simulink model "CML_Iso_Force_Production"  (R2015a)
settings: Solver=ode4  SolverMode=MultiTasking  StartTime=0.0  StopTime=inf  FixedStep=BKIN_STEP_TIME  RelTol=1e-3
StartFcn:
  |  warndlg('Dexterit-E models cannot run under simulation. Please compile your model and run it from within Dexterit-E.');set_param(bdroot,'SimulationCommand','stop')
model workspace (MAT data in the model file):
  BKIN_STEP_TIME = 0.00025
  col_x = 1
  col_y = 2
  VRAD = 3
  COLOR = 4
  TARGET_COL = 2
  BKIN_KINEMATIC_FRAME_SIZE = 400
  E_NO_EVENT = 0
  K_START_TGT = 1
  INIT_DUR = 5
  TP_ITI = 9
  K_JOINT_ASSESSED = 2
  TEXT1 = 5
  TEXT2 = 6
  HEIGHT = 7
  STROKE_WIDTH = 8
  GOAL_F_PCT = 3
  DO_FDBK = 8
  MAX_MOVE_TIME = 7
  MIN_FORCE = 4
  E_TEST_MVC = 1
  E_HOLD_MVC = 3
  E_EOT = 10
  E_FORCE_TRIAL = 11
  E_HOLD_FORCE = 13
  K_BAR_TGT = 3
  K_MVC_TEXT_TGT = 4
  E_INIT_FORCE = 12
  E_SET_MVC = 2
  K_MVC = 5
  TRIAL_TYPE = 1
  HOLD_TIME = 6
  E_ERROR_TRIAL = 5
  E_ACCEPT_MVC = 6
  ACCEPT_MVC = 2
  REJECT_MVC = 3
  E_CHECK_MVC = 4
  E_REJECT_MVC = 5
libraries: Video x5, slrtlib x5, General x3, KINARM_IO x2, simulink x2, KINARM_loads x2, KINARM_general x1, xpcnilib x1
CloseFcn:
  | rtwprivate ssgencode ModelCloseRequest b2lab2d
settings Model: ModifiedComment=chris -- Wed Feb 16 09:18:30 2005 -- Version 1.1384  ExtModeArmWhenConnect=off  ExtModeLogAll=off  LastModifiedBy=User
settings SolverCC: EnableConcurrentExecution=on  AutoInsertRateTranBlk=on
settings DataIOCC: LimitDataPoints=off  SignalLoggingSaveFormat=ModelDataLogs  SaveOutput=off  SaveTime=off  SignalLoggingName=sigsOut
settings OptimizationCC: BlockReduction=off  BooleanDataType=off  OptimizeBlockIOStorage=off  BufferReuse=off  GlobalBufferReuse=off  ExpressionFolding=off  ExpressionDepthLimit=2147483647  LocalBlockOutputs=off  InitFltsAndDblsToZero=on
settings DebuggingCC: SaveWithParameterizedLinksMsg=none  UnderspecifiedInitializationDetection=Classic  MergeDetectMultiDrivingBlocksExec=none  SignalResolutionControl=TryResolveAllWithWarning  MultiTaskDSMMsg=warning  FcnCallInpInsideContextMsg=UseLocalSettings  StateNameClashWarn=warning  StrictBusMsg=ErrorOnBusTreatedAsVector
settings HardwareCC: ProdIntDivRoundTo=Zero  ProdEndianess=LittleEndian  ProdLongLongMode=on  ProdHWDeviceType=Generic->32-bit x86 compatible  TargetHWDeviceType=32-bit Generic
settings SFSimCC: SimParseCustomCode=off
settings RTWCC: SystemTargetFile=slrt.tlc  TemplateMakefile=slrt_default_tmf  Description=Simulink Real-Time  RTWCompilerOptimization=on
settings CodeAppCC: MaxIdLength=63
settings SimulinkRealTimeCC: TargetFcnLib=ansi_tfl_tmw.mat  GeneratePreprocessorConditionals=Disable all  xPCisDownloadable=off

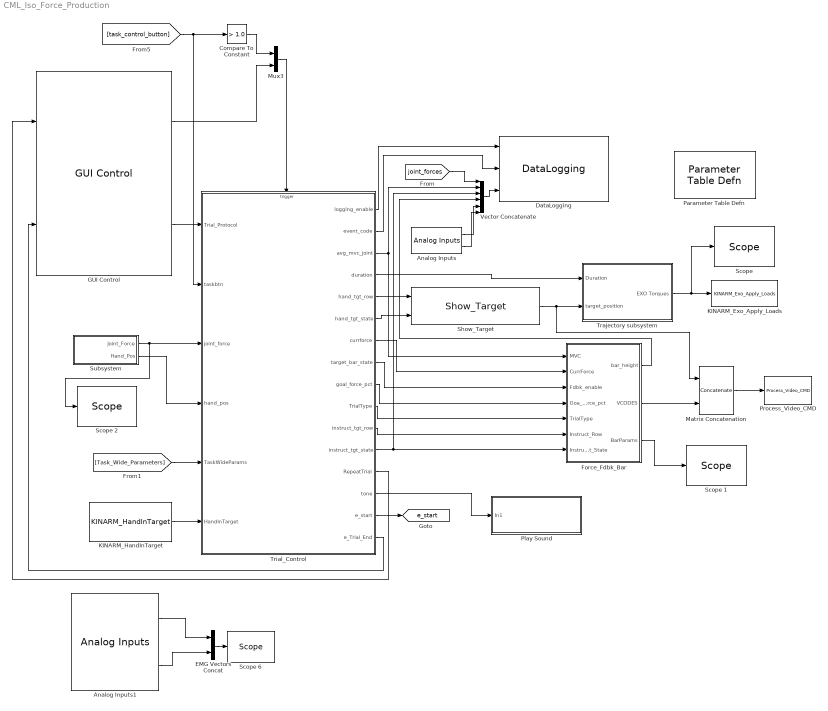
== system CML_Iso_Force_Production ==
  Analog Inputs : KINARM_IO/Analog Inputs  channel=[18:19]  range=[5]  coupling=[0]  scantime6071e=1.28e-5  scantime6229=5e-6  sampletime=0.001  slot=-1  oscantime6071e=0
  Analog Inputs1 : KINARM_IO/Analog Inputs  channel=[18:19]  range=[5]  coupling=[0]  scantime6071e=1.28e-5  scantime6229=5e-6  sampletime=0.001  slot=-1  oscantime6071e=0
  Compare To Constant : simulink/Logic and Bit Operations/Compare To Constant  relop=>  const=1.0  OutDataTypeStr=boolean
  DataLogging : General/DataLogging  log_event_codes=on  log_analog_inputs=on  show_time_remaining=off  ecat_include=on
      link override Poll KINARM/EPTorqueCMD: GotoTag=KINARMEPTorqueCMD
      link override Poll KINARM/TorqueCMD: GotoTag=KINARMTorqueCMD
  EMG Vectors Concat : Concatenate
  Force_Fdbk_Bar : Subsystem
  GUI Control : General/GUI Control  task_version=1.0  show_repeat_trial_flag=on  use_custom_tp=off  target_type_str=Circle  Target_Type=1  XYcols=[1 2]  Vcols=3  Lcols=4  indices_padding=[0 0 0 0;0 0 0 0]  target_table_rows=64  load_table_rows=20  tp_table_rows=100
  KINARM_Exo_Apply_Loads : KINARM_loads/KINARM_Exo_Apply_Loads  up_duration=1000  down_duration=1000  max_torque=10  limit_motors=off
  KINARM_HandInTarget : KINARM_general/KINARM_HandInTarget  use_dominant_hand=on  target_type=Circle  num_states=1  attribcol1=[VRAD]  attribcol2=[0]  attribcol3=[0]  attribcol4=[0]  attribcol5=[0]
  Matrix Concatenation : Concatenate  Mode=Multidimensional array
  Mux3 : Mux  Inputs=2
  Parameter Table Defn : General/Parameter Table Defn  ShowInLibBrowser=0
  Play Sound : Subsystem
  Process_Video_CMD : Video/Process_Video_CMD  video_delay=0
  "Scope " : slrtlib/Displays and Logging/Scope   scopeno=1  scopetype=Target  autostart=on  viewmode=Numerical  formatstr='%15.6f'  grid=on  ylimits=[0,0]  nosamples=250  noprepostsamples=0  interleave=1  triggermode=FreeRun  triggersignal=1  trigsignalfromport=off  triggerlevel=0.0  triggerslope=Either  triggerscope=1  triggersample=0  filename=data.dat  mode=Lazy  writesize=512  autorestart=off  dynamicfilemode=off  maxwritefilesize=512*1024^2
  Scope 1 : slrtlib/Displays and Logging/Scope   scopeno=2  scopetype=Target  autostart=on  viewmode=Numerical  formatstr='%15.6f'  grid=on  ylimits=[0,0]  nosamples=250  noprepostsamples=0  interleave=1  triggermode=FreeRun  triggersignal=1  trigsignalfromport=off  triggerlevel=0.0  triggerslope=Either  triggerscope=1  triggersample=0  filename=data.dat  mode=Lazy  writesize=512  autorestart=off  dynamicfilemode=off  maxwritefilesize=512*1024^2
  Scope 2 : slrtlib/Displays and Logging/Scope   scopeno=3  scopetype=Target  autostart=on  viewmode=Numerical  formatstr='%15.6f'  grid=on  ylimits=[0,0]  nosamples=250  noprepostsamples=0  interleave=1  triggermode=FreeRun  triggersignal=1  trigsignalfromport=off  triggerlevel=0.0  triggerslope=Either  triggerscope=1  triggersample=0  filename=data.dat  mode=Lazy  writesize=512  autorestart=off  dynamicfilemode=off  maxwritefilesize=512*1024^2
  Scope 6 : slrtlib/Displays and Logging/Scope   scopeno=4  scopetype=Target  autostart=on  viewmode=Numerical  formatstr='%15.6f'  grid=on  ylimits=[0,0]  nosamples=250  noprepostsamples=0  interleave=1  triggermode=FreeRun  triggersignal=1  trigsignalfromport=off  triggerlevel=0.0  triggerslope=Either  triggerscope=1  triggersample=0  filename=data.dat  mode=Lazy  writesize=512  autorestart=off  dynamicfilemode=off  maxwritefilesize=512*1024^2
  Show_Target : Video/Show_Target  target_type=Circle  num_states=1  attribcol1=[COLOR 0 0 VRAD]  attribcol2=[0 0 0 0]  attribcol3=[0 0 0 0]  attribcol4=[0 0 0 0]  attribcol5=[0 0 0 0]  stateindices_padding=[0 0 0 0 0 0 0;0 0 0 0 0 0 0;0 0 0 0 0 0 0;0 0 0 0 0 0 0;0 0 0 0 0 0 0]  source=dialog  opacity=100  target_display=Both subject and operator displays  num_col=4
  Subsystem : Subsystem
  Trajectory subsystem : Subsystem
  Trial_Control : Stateflow chart  TreatAsAtomicUnit=on
  Vector Concatenate : Concatenate  NumInputs=6
  tag scope: e_start=global
  wires:
  Show_Target/1 -> Matrix Concatenation/1, Trajectory subsystem/2(target_position)
  Trial_Control/16(e_Trial_End) -> GUI Control/2
  GUI Control/1 -> Mux3/2
  Trial_Control/6(hand_tgt_state) -> Show_Target/2
  Trial_Control/5(hand_tgt_row) -> Show_Target/1
  Matrix Concatenation/1 -> Process_Video_CMD/1
  GUI Control/2 -> Trial_Control/1(Trial_Protocol)
  Trial_Control/1(logging_enable) -> DataLogging/1
  Trial_Control/4(duration) -> Trajectory subsystem/1(Duration)
  Trajectory subsystem/1(EXO Torques) -> "Scope "/1, KINARM_Exo_Apply_Loads/1
  Trial_Control/15(e_start) -> [e_start]
  [joint_forces] -> Vector Concatenate/1
  Vector Concatenate/1 -> DataLogging/3
  Analog Inputs/1 -> Vector Concatenate/5
  Subsystem/1(Joint_Force) -> Scope 2/1, Trial_Control/3(joint_force)
  Subsystem/2(Hand_Pos) -> Trial_Control/4(hand_pos)
  [Task_Wide_Parameters] -> Trial_Control/5(TaskWideParams)
  Trial_Control/11(instruct_tgt_row) -> Force_Fdbk_Bar/6(Instruct_Row)
  Trial_Control/12(instruct_tgt_state) -> Force_Fdbk_Bar/7(Instruct_State), Vector Concatenate/3
  Trial_Control/3(avg_mvc_joint) -> Force_Fdbk_Bar/1(MVC), Vector Concatenate/2
  Force_Fdbk_Bar/2(VCODES) -> Matrix Concatenation/2
  Trial_Control/8(target_bar_state) -> Force_Fdbk_Bar/3(Fdbk_enable)
  Trial_Control/7(currforce) -> Force_Fdbk_Bar/2(CurrForce)
  Trial_Control/9(goal_force_pct) -> Force_Fdbk_Bar/4(Goa_force_pct)
  Force_Fdbk_Bar/1(bar_height) -> Vector Concatenate/4
  Force_Fdbk_Bar/3(BarParams) -> Scope 1/1
  Trial_Control/2(event_code) -> DataLogging/2
  Trial_Control/10(TrialType) -> Force_Fdbk_Bar/5(TrialType)
  KINARM_HandInTarget/1 -> Trial_Control/6(HandInTarget)
  Trial_Control/14(tone) -> Play Sound/1(In1)
  Trial_Control/13(RepeatTrial) -> GUI Control/1
  [task_control_button] -> Compare To Constant/1, Trial_Control/2(taskbtn)
  Compare To Constant/1 -> Mux3/1
  Mux3/1 -> Trial_Control/Trigger
  EMG Vectors Concat/1 -> Scope 6/1
  Analog Inputs1/1 -> EMG Vectors Concat/1
  Analog Inputs1/2 -> EMG Vectors Concat/2
  Analog Inputs/2 -> Vector Concatenate/6

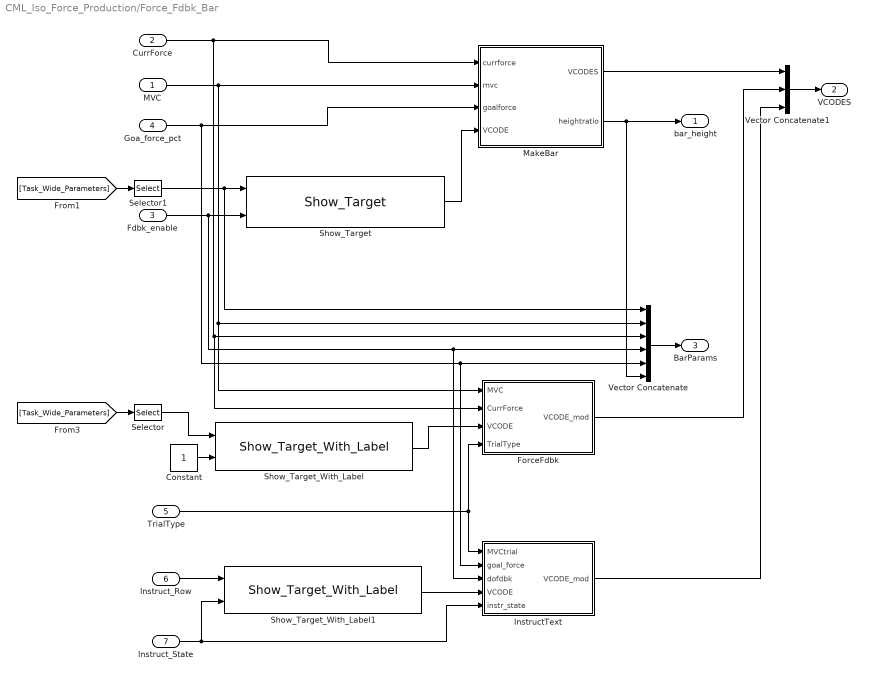
== system CML_Iso_Force_Production/Force_Fdbk_Bar ==
  MVC : Inport
  CurrForce : Inport  Port=2
  Fdbk_enable : Inport  Port=3
  Goa_force_pct : Inport  Port=4
  TrialType : Inport  Port=5
  Instruct_Row : Inport  Port=6
  Instruct_State : Inport  Port=7
  Constant : Constant
  ForceFdbk : MATLAB Function  TreatAsAtomicUnit=on
  InstructText : MATLAB Function  TreatAsAtomicUnit=on
  MakeBar : MATLAB Function  TreatAsAtomicUnit=on
  Selector : Selector  InputPortWidth=50  Indices=[K_MVC_TEXT_TGT]
  Selector1 : Selector  InputPortWidth=50  Indices=[K_BAR_TGT]
  Show_Target : Video/Show_Target  target_type=Rectangle  num_states=1  attribcol1=[COLOR 0 STROKE_WIDTH VRAD HEIGHT 0]  attribcol2=[0 0 0 0 0 0]  attribcol3=[0 0 0 0 0 0]  attribcol4=[0 0 0 0 0 0]  attribcol5=[0 0 0 0 0 0]  stateindices_padding=[0 0 0 0 0;0 0 0 0 0;0 0 0 0 0;0 0 0 0 0;0 0 0 0 0]  source=dialog  opacity=100  target_display=Both subject and operator displays  num_col=6
  Show_Target_With_Label : Video/Show_Target_With_Label  target_type=Rectangle  num_states=1  attribcol1=[0 0 0 VRAD HEIGHT 0 TEXT1 COLOR HEIGHT]  attribcol2=[0 0 0 0 0 0 0 0 0]  attribcol3=[0 0 0 0 0 0 0 0 0]  attribcol4=[0 0 0 0 0 0 0 0 0]  attribcol5=[0 0 0 0 0 0 0 0 0]  stateindices_padding=[0 0;0 0;0 0;0 0;0 0]  source=dialog  opacity=100  target_display=Operator display only
  Show_Target_With_Label1 : Video/Show_Target_With_Label  target_type=Rectangle  num_states=2  attribcol1=[0 0 0 VRAD HEIGHT 0 TEXT1 COLOR HEIGHT]  attribcol2=[0 0 0 VRAD HEIGHT 0 TEXT2 COLOR HEIGHT]  attribcol3=[0 0 0 0 0 0 0 0 0]  attribcol4=[0 0 0 0 0 0 0 0 0]  attribcol5=[0 0 0 0 0 0 0 0 0]  stateindices_padding=[0 0;0 0;0 0;0 0;0 0]  source=dialog  opacity=100  target_display=Both subject and operator displays
  Vector Concatenate : Concatenate  NumInputs=6
  Vector Concatenate1 : Concatenate  NumInputs=3  Mode=Multidimensional array
  bar_height : Outport
  VCODES : Outport  Port=2
  BarParams : Outport  Port=3
  wires:
  Fdbk_enable/1 -> InstructText/3(dofdbk), Vector Concatenate/4, Show_Target/2
  Selector1/1 -> Vector Concatenate/1, Show_Target/1
  CurrForce/1 -> ForceFdbk/2(CurrForce), Vector Concatenate/3, MakeBar/1(currforce)
  MVC/1 -> ForceFdbk/1(MVC), Vector Concatenate/2, MakeBar/2(mvc)
  Show_Target/1 -> MakeBar/4(VCODE)
  MakeBar/1(VCODES) -> Vector Concatenate1/1
  Goa_force_pct/1 -> Vector Concatenate/5, InstructText/2(goal_force), MakeBar/3(goalforce)
  MakeBar/2(heightratio) -> Vector Concatenate/6, bar_height/1
  Vector Concatenate/1 -> BarParams/1
  Constant/1 -> Show_Target_With_Label/2
  Show_Target_With_Label/1 -> ForceFdbk/3(VCODE)
  ForceFdbk/1(VCODE_mod) -> Vector Concatenate1/2
  Vector Concatenate1/1 -> VCODES/1
  TrialType/1 -> ForceFdbk/4(TrialType), InstructText/1(MVCtrial)
  Selector/1 -> Show_Target_With_Label/1
  [Task_Wide_Parameters] -> Selector/1
  Show_Target_With_Label1/1 -> InstructText/4(VCODE)
  Instruct_Row/1 -> Show_Target_With_Label1/1
  Instruct_State/1 -> InstructText/5(instr_state), Show_Target_With_Label1/2
  InstructText/1(VCODE_mod) -> Vector Concatenate1/3
  [Task_Wide_Parameters] -> Selector1/1

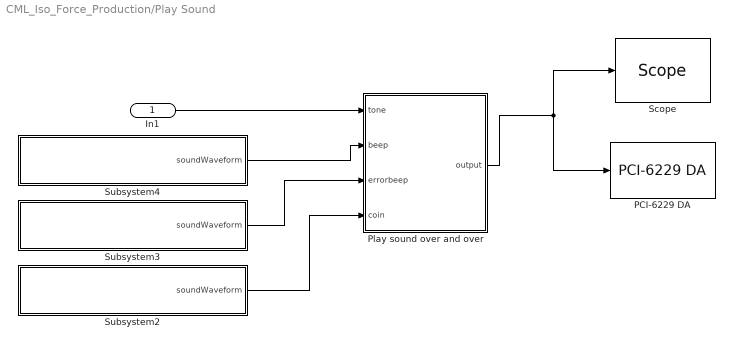
== system CML_Iso_Force_Production/Play Sound ==
  In1 : Inport
  PCI-6229 DA : xpcnilib/D//A/M Series/PCI-6229 DA  channel=[1]  reset=[1]  initValue=[0]  sampletime=-1  slot=-1
  Play sound over and over : MATLAB Function  TreatAsAtomicUnit=on
  "Scope " : slrtlib/Displays and Logging/Scope   scopeno=5  scopetype=Target  autostart=on  viewmode=Graphical redraw  formatstr='%15.6f'  grid=on  ylimits=[0,0]  nosamples=4000  noprepostsamples=0  interleave=1  triggermode=FreeRun  triggersignal=1  trigsignalfromport=off  triggerlevel=0.0  triggerslope=Either  triggerscope=1  triggersample=0  filename=data.dat  mode=Lazy  writesize=512  autorestart=off  dynamicfilemode=off  maxwritefilesize=512*1024^2
  Subsystem2 : Subsystem  mask(Load Waveform Into Variable){fileName=coin.mat}
      mask prompts: fileName "Name of .mat Data File (must be in current directory)"
      mask help: This block will load the .MAT file specified in the dialog, and put the first variable into a GoTo called 'soundWaveform'.
      mask init:
      | filenameFromMask = get_param(gcb, 'fileName');
      | 
      | try 
      | 	dataFromFile = load(filenameFromMask);
      | 	names = fieldnames(dataFromFile);
      | 	soundDataFromFile = dataFromFile.(names{1});
      | 	display(['Sound waveform from file ''' filenameFromMask ''' loaded.']);
      | catch ME
      | 	display(ME.message)
      | end
      mask Help:
      | Enter the name a .MAT file containing a single vector or matrix. The .MAT file must be located in the current directory.
      | 
      | The first variable from the .MAT file will be put into a Goto called 'soundWaveform'.
      mask Display: disp(['Load waveform from ''' filenameFromMask ''''])
  Subsystem3 : Subsystem  mask(Load Waveform Into Variable){fileName=errorbeep.mat}
      mask prompts: fileName "Name of .mat Data File (must be in current directory)"
      mask help: This block will load the .MAT file specified in the dialog, and put the first variable into a GoTo called 'soundWaveform'.
      mask init: same as CML_Iso_Force_Production/Play Sound/Subsystem2
      mask Help:
      | Enter the name a .MAT file containing a single vector or matrix. The .MAT file must be located in the current directory.
      | 
      | The first variable from the .MAT file will be put into a Goto called 'soundWaveform'.
      mask Display: disp(['Load waveform from ''' filenameFromMask ''''])
  Subsystem4 : Subsystem  mask(Load Waveform Into Variable){fileName=startbeep.mat}
      mask prompts: fileName "Name of .mat Data File (must be in current directory)"
      mask help: This block will load the .MAT file specified in the dialog, and put the first variable into a GoTo called 'soundWaveform'.
      mask init: same as CML_Iso_Force_Production/Play Sound/Subsystem2
      mask Help:
      | Enter the name a .MAT file containing a single vector or matrix. The .MAT file must be located in the current directory.
      | 
      | The first variable from the .MAT file will be put into a Goto called 'soundWaveform'.
      mask Display: disp(['Load waveform from ''' filenameFromMask ''''])
  wires:
  Play sound over and over/1(output) -> PCI-6229 DA/1, "Scope "/1
  Subsystem3/1(soundWaveform) -> Play sound over and over/3(errorbeep)
  Subsystem4/1(soundWaveform) -> Play sound over and over/2(beep)
  In1/1 -> Play sound over and over/1(tone)
  Subsystem2/1(soundWaveform) -> Play sound over and over/4(coin)

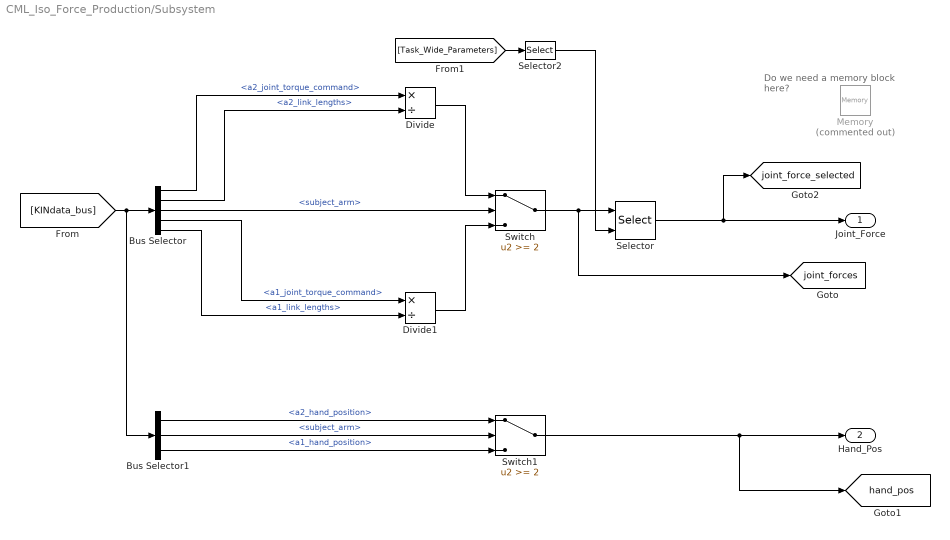
== system CML_Iso_Force_Production/Subsystem ==
  note: Do we need a memory block here?
  Bus Selector : BusSelector  OutputSignals=Robot2.a2_joint_torque_command,Robot2.a2_link_lengths,KINDataGeneral.subject_arm,Robot1.a1_joint_torque_command,Robot1.a1_link_lengths
  Bus Selector1 : BusSelector  OutputSignals=Robot2.a2_hand_position,KINDataGeneral.subject_arm,Robot1.a1_hand_position
  Divide : Product  Inputs=*/
  Divide1 : Product  Inputs=*/
  Memory : Memory  Commented=on
  Selector : Selector  InputPortWidth=2  IndexOptions=Index vector (port)  Indices=[1 3]
  Selector2 : Selector  InputPortWidth=50  Indices=[K_JOINT_ASSESSED]
  Switch : Switch  Threshold=2
  Switch1 : Switch  Threshold=2
  Joint_Force : Outport
  Hand_Pos : Outport  Port=2
  tag scope: hand_pos=global, joint_force_selected=global, joint_forces=global
  wires:
  [KINdata_bus] -> Bus Selector1/1, Bus Selector/1
  Bus Selector/3 -> Switch/2  "<subject_arm>"
  Divide/1 -> Switch/1
  Divide1/1 -> Switch/3
  Bus Selector/1 -> Divide/1  "<a2_joint_torque_command>"
  Bus Selector/2 -> Divide/2  "<a2_link_lengths>"
  Bus Selector/4 -> Divide1/1  "<a1_joint_torque_command>"
  Bus Selector/5 -> Divide1/2  "<a1_link_lengths>"
  Bus Selector1/1 -> Switch1/1  "<a2_hand_position>"
  Bus Selector1/2 -> Switch1/2  "<subject_arm>"
  Bus Selector1/3 -> Switch1/3  "<a1_hand_position>"
  Switch/1 -> Selector/1, [joint_forces]
  Selector2/1 -> Selector/2
  Switch1/1 -> [hand_pos], Hand_Pos/1
  Selector/1 -> [joint_force_selected], Joint_Force/1
  [Task_Wide_Parameters] -> Selector2/1

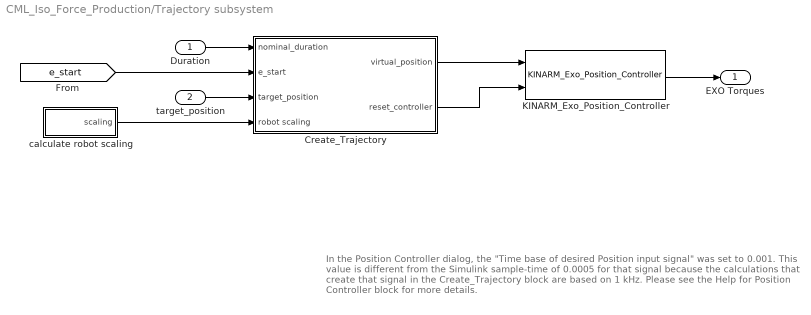
== system CML_Iso_Force_Production/Trajectory subsystem ==
  note: In the Position Controller dialog, the "Time base of desired Position input signal" was set to 0.001.
      | This value is different from the Simulink sample-time of 0.0005 for that signal because the calculations
      | that create that signal in the Create_Trajectory block are based on 1 kHz. Please see the Help for
      | Position Controller block for more details.
  Duration : Inport
  target_position : Inport  Port=2
  Create_Trajectory : Subsystem
  KINARM_Exo_Position_Controller : KINARM_loads/KINARM_Exo_Position_Controller  use_dom_hand=on  KINARM_Type=Human  inertias_for_FF=KINARM robot  angles_or_XY=End-point (global x/y)  sample_time=0.001
  calculate robot scaling : Subsystem
  EXO Torques : Outport
  wires:
  Create_Trajectory/2(reset_controller) -> KINARM_Exo_Position_Controller/2
  Create_Trajectory/1(virtual_position) -> KINARM_Exo_Position_Controller/1
  KINARM_Exo_Position_Controller/1 -> EXO Torques/1
  target_position/1 -> Create_Trajectory/3(target_position)
  Duration/1 -> Create_Trajectory/1(nominal_duration)
  [e_start] -> Create_Trajectory/2(e_start)
  calculate robot scaling/1(scaling) -> Create_Trajectory/4(robot scaling)

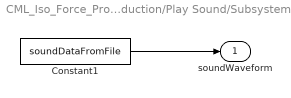
== system CML_Iso_Force_Production/Play Sound/Subsystem2 ==
  Constant1 : Constant  Value=soundDataFromFile
  soundWaveform : Outport
  wires:
  Constant1/1 -> soundWaveform/1

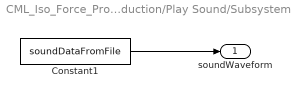
== system CML_Iso_Force_Production/Play Sound/Subsystem3 ==
  Constant1 : Constant  Value=soundDataFromFile
  soundWaveform : Outport
  wires:
  Constant1/1 -> soundWaveform/1

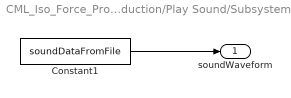
== system CML_Iso_Force_Production/Play Sound/Subsystem4 ==
  Constant1 : Constant  Value=soundDataFromFile
  soundWaveform : Outport
  wires:
  Constant1/1 -> soundWaveform/1

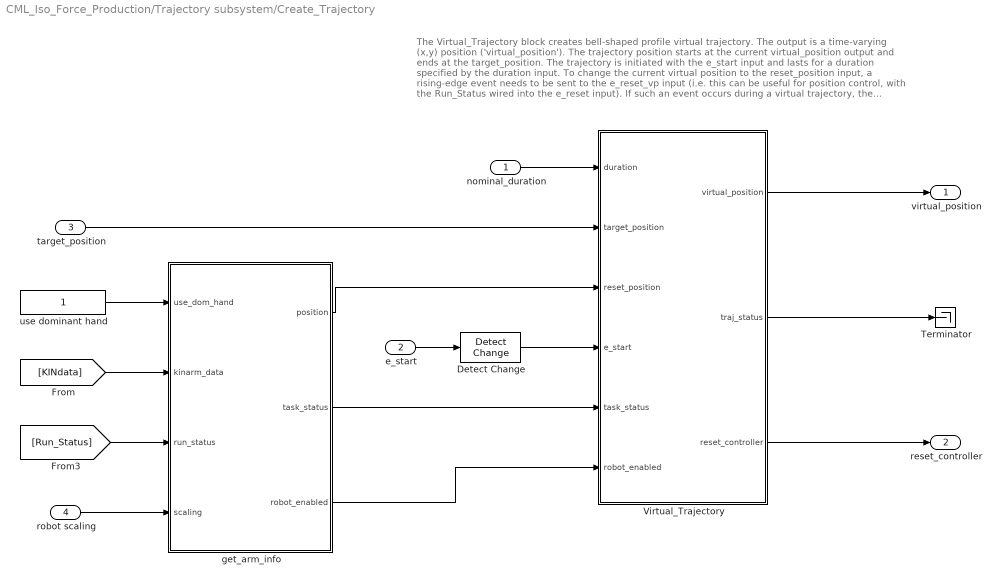
== system CML_Iso_Force_Production/Trajectory subsystem/Create_Trajectory ==
  note: The Virtual_Trajectory block creates bell-shaped profile virtual trajectory.
      | The output is a time-varying (x,y) position ('virtual_position').
      |
      | The trajectory position starts at the current virtual_position output and ends at the target_position.
      | The trajectory is initiated with the e_start input and lasts for a duration specified by the duration input.
      |
      | To change the current virtual position to the reset_position input, a rising-edge event needs to be sent to the e_reset_vp input
      | (i.e. this can be useful for position control, with the Run_Status wired into the e_reset input).
      | If such an event occurs during a virtual trajectory, the trajectory is halted immediately.
  nominal_duration : Inport
  e_start : Inport  Port=2
  target_position : Inport  Port=3
  robot scaling : Inport  Port=4
  Detect Change : simulink/Logic and Bit Operations/Detect Change  vinit=0  InputProcessing=Inherited  OutDataTypeStr=uint8
  Terminator : Terminator
  Virtual_Trajectory : Subsystem
  get_arm_info : MATLAB Function  TreatAsAtomicUnit=on
  use dominant hand : Constant
  virtual_position : Outport
  reset_controller : Outport  Port=2
  wires:
  Virtual_Trajectory/1(virtual_position) -> virtual_position/1
  nominal_duration/1 -> Virtual_Trajectory/1(duration)
  e_start/1 -> Detect Change/1
  target_position/1 -> Virtual_Trajectory/2(target_position)
  Detect Change/1 -> Virtual_Trajectory/4(e_start)
  use dominant hand/1 -> get_arm_info/1(use_dom_hand)
  [KINdata] -> get_arm_info/2(kinarm_data)
  get_arm_info/1(position) -> Virtual_Trajectory/3(reset_position)
  Virtual_Trajectory/3(reset_controller) -> reset_controller/1
  get_arm_info/2(task_status) -> Virtual_Trajectory/5(task_status)
  get_arm_info/3(robot_enabled) -> Virtual_Trajectory/6(robot_enabled)
  [Run_Status] -> get_arm_info/3(run_status)
  Virtual_Trajectory/2(traj_status) -> Terminator/1
  robot scaling/1 -> get_arm_info/4(scaling)

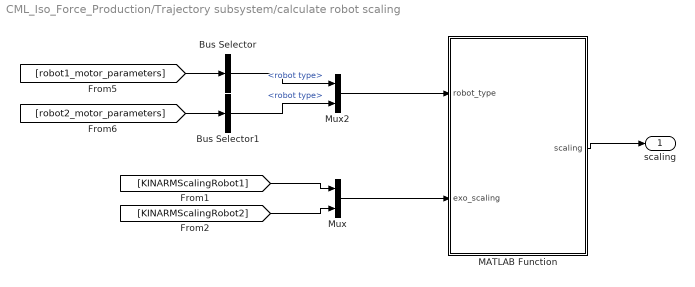
== system CML_Iso_Force_Production/Trajectory subsystem/calculate robot scaling ==
  Bus Selector : BusSelector  OutputSignals=robot type
  Bus Selector1 : BusSelector  OutputSignals=robot type
  MATLAB Function : MATLAB Function  TreatAsAtomicUnit=on
  Mux : Mux  Inputs=2
  Mux2 : Mux  Inputs=2
  scaling : Outport
  wires:
  [KINARMScalingRobot1] -> Mux/1
  [KINARMScalingRobot2] -> Mux/2
  Mux/1 -> MATLAB Function/2(exo_scaling)
  Mux2/1 -> MATLAB Function/1(robot_type)
  MATLAB Function/1(scaling) -> scaling/1
  [robot2_motor_parameters] -> Bus Selector1/1
  Bus Selector1/1 -> Mux2/2  "<robot type>"
  Bus Selector/1 -> Mux2/1  "<robot type>"
  [robot1_motor_parameters] -> Bus Selector/1

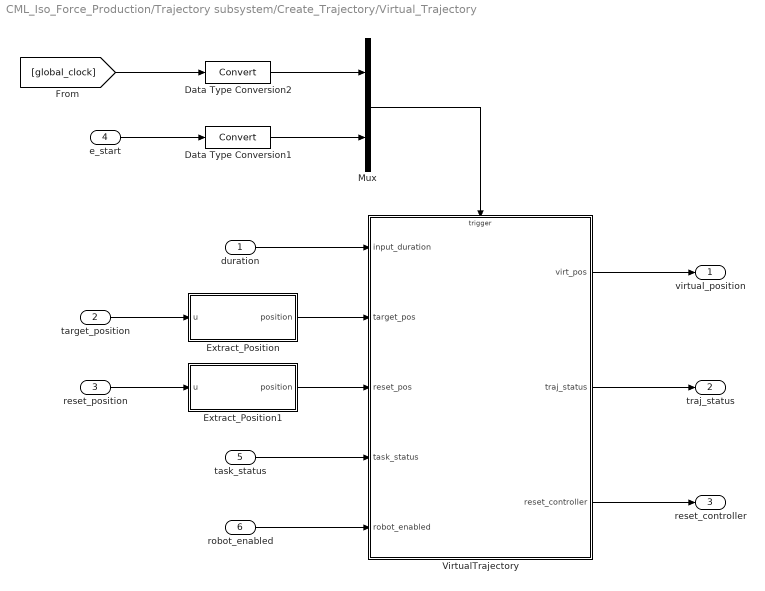
== system CML_Iso_Force_Production/Trajectory subsystem/Create_Trajectory/Virtual_Trajectory ==
  duration : Inport
  target_position : Inport  Port=2
  reset_position : Inport  Port=3
  e_start : Inport  Port=4
  task_status : Inport  Port=5
  robot_enabled : Inport  Port=6
  Data Type Conversion1 : DataTypeConversion
  Data Type Conversion2 : DataTypeConversion
  Extract_Position : MATLAB Function  TreatAsAtomicUnit=on
  Extract_Position1 : MATLAB Function  TreatAsAtomicUnit=on
  Mux : Mux  Inputs=2
  VirtualTrajectory : Stateflow chart  TreatAsAtomicUnit=on
  virtual_position : Outport
  traj_status : Outport  Port=2
  reset_controller : Outport  Port=3
  wires:
  e_start/1 -> Data Type Conversion1/1
  target_position/1 -> Extract_Position/1(u)
  [global_clock] -> Data Type Conversion2/1
  Mux/1 -> VirtualTrajectory/Trigger
  duration/1 -> VirtualTrajectory/1(input_duration)
  VirtualTrajectory/1(virt_pos) -> virtual_position/1
  Extract_Position/1(position) -> VirtualTrajectory/2(target_pos)
  reset_position/1 -> Extract_Position1/1(u)
  Data Type Conversion2/1 -> Mux/1
  VirtualTrajectory/2(traj_status) -> traj_status/1
  robot_enabled/1 -> VirtualTrajectory/5(robot_enabled)
  task_status/1 -> VirtualTrajectory/4(task_status)
  Data Type Conversion1/1 -> Mux/2
  Extract_Position1/1(position) -> VirtualTrajectory/3(reset_pos)
  VirtualTrajectory/3(reset_controller) -> reset_controller/1

== stateflow chart CML_Iso_Force_Production/Trial_Control ==
  settings: sampleTime=0.001
  state init/
    //bring the hand to the start position
    mvc_joint = 0;
    avg_mvc_joint = TaskWideParams[K_MVC];
    n_mvc = 1*(avg_mvc_joint>1e-4);
    hand_tgt_row = TaskWideParams[K_START_TGT];
    hand_tgt_state = 1;
    instruct_tgt_row = 0;
    instruct_tgt_state = 0;
    duration = 3000;
  state MovToStart/
    ITI = Trial_Protocol[TP_ITI];
    TrialType = Trial_Protocol[TRIAL_TYPE];
    RepeatTrial = 0;
    instruct_tgt_state = 0;
    target_bar_state = 0;
    currforce = 0;
    tone = 0;
    e_start;
  state Main_Trial
    state InitMVC/
      event_code = E_TEST_MVC;
      logging_enable = 1;
      duration = 1;
      instruct_tgt_row = Trial_Protocol[TARGET_COL];
      instruct_tgt_state = 1;
      min_force = Trial_Protocol[MIN_FORCE];
      tmpforce = 0;
      tmpcounter = 0;
      iforce = 0;
      maxforce = min_force;
      hold_time = Trial_Protocol[HOLD_TIME];
      max_move_time = Trial_Protocol[MAX_MOVE_TIME];
      tick = 0;
      tone = 1;
    state InitForceTrial/
      event_code = E_FORCE_TRIAL;
      logging_enable = 1;
      duration = 1;
      instruct_tgt_row = Trial_Protocol[TARGET_COL];
      instruct_tgt_state = 1;
      tmpforce = 0;
      tmpcounter = 0;
      iforce = 0;
      maxforce = 0;
      goal_force_pct = Trial_Protocol[GOAL_F_PCT];
      goal_force = avg_mvc_joint*(goal_force_pct/100.0);
      target_bar_state = Trial_Protocol[DO_FDBK];
      min_force = Trial_Protocol[MIN_FORCE];
      force_thresh = min_force;
      force_thresh += force_thresh*(target_bar_state == 0); //if no feedback, relax the criterion
      hold_time = Trial_Protocol[HOLD_TIME];
      max_move_time = Trial_Protocol[MAX_MOVE_TIME];
      tick = 0;
    state SetMVC/
      event_code = E_SET_MVC;
      tmpcounter = 0;
      tmp_forcehist = 0;
      iforce = 0;
      during: //check and update the estimated mvc
      tick++;
      currforce = joint_force;
      [maxforce,iforce,tmp_forcehist] = calcmvc(tmp_forcehist,iforce,joint_force)
    state HoldMVC/
      event_code = E_HOLD_MVC;
      tone = 0;
      during: //check and update the estimated mvc
      tick++;
      tmpcounter++;
      currforce = joint_force;
    state ApplyForce/
      event_code = E_INIT_FORCE;
      during:
      maxforce = joint_force;
      currforce = joint_force;
      tmpcounter = 0;
      tick++;
    state WaitAcceptMVC/
      event_code = E_CHECK_MVC;
      currforce = maxforce;
      instruct_tgt_state = 2;
      tone = 1;
    state HoldAppliedForce/
      event_code = E_HOLD_FORCE;
      during:
      maxforce = joint_force;
      currforce = joint_force;
      tmpcounter++;
      tick++;
    state AcceptMVC/
      event_code = E_ACCEPT_MVC;
      //record the MVC on this trial if desired
      mvc_joint += maxforce; %*(tmpcounter >= force_hold_time);
      n_mvc += 1; %*(tmpcounter >= force_hold_time);
      avg_mvc_joint = mvc_joint/n_mvc;
      currforce = avg_mvc_joint;
    state EndMVC1/
      event_code = E_EOT;
    state EndOfTrial/
      event_code = E_EOT;
      instruct_tgt_state = 2;
    (junction 75) -> InitMVC [order 2] : [TrialType == 1]
    (junction 75) -> InitForceTrial [order 1] : [TrialType == 2]/
    InitMVC -> SetMVC : [(joint_force > min_force) && after(1, e_clk)]
    InitForceTrial -> ApplyForce : [(joint_force > min_force) && after(1, e_clk)]
    SetMVC -> HoldMVC [order 1] : [abs(joint_force - maxforce) < min_force]
    HoldMVC -> SetMVC [order 2] : [abs(joint_force-maxforce) > min_force]
    HoldMVC -> WaitAcceptMVC [order 1] : [(tmpcounter >= hold_time)]
    SetMVC -> WaitAcceptMVC [order 2] : [(tick > max_move_time) ]
    ApplyForce -> HoldAppliedForce : [joint_force > goal_force]
    HoldAppliedForce -> ApplyForce [order 1] : [abs(joint_force - goal_force) > force_thresh]/
        | //apply the force threshold on either side of the goal
    WaitAcceptMVC -> AcceptMVC [order 1] : [taskbtn == 2]
    WaitAcceptMVC -> EndMVC1 [order 2] : [taskbtn == 3]/
        | RepeatTrial = 1;
        | event_code = E_REJECT_MVC;
    HoldAppliedForce -> EndOfTrial [order 2] : [(tmpcounter > hold_time) || (tick > max_move_time) ]
    AcceptMVC -> EndMVC1
    EndMVC1 -> (junction 111) : [joint_force <= min_force]
    EndOfTrial -> (junction 111) : [joint_force <= min_force]
  state MeasureMVC1/ [commented out]
    event_code = E_HOLD_MVC;
    during: //check and update the estimated mvc
    [tmpforce, tmpcounter, iforce, maxforce] = update_mvc(tmpforce,joint_force,tmpcounter, iforce, maxforce, min_force);
    tick++;
  state Inter_Trial_State/
    e_Trial_End
    duration = Trial_Protocol[INIT_DUR];
  state WaitForFlagToSet
  state EndMVC/ [commented out]
    event_code = E_EOT;
    //record the MVC on this trial if it was a good trial (i.e., it didn't time out)
    mvc_joint += maxforce;
    n_mvc += 1;
    avg_mvc_joint = mvc_joint/n_mvc;
    currforce = avg_mvc_joint;
    instruct_tgt_state = 2;
  (default) -> init
  init -> (junction 85)
  MovToStart -> (junction 75) : [after(duration, e_clk) && HandInTarget[hand_tgt_row]]/
      | //hand_tgt_state = 0;
  (junction 85) -> MovToStart
  Inter_Trial_State -> (junction 85)
  WaitForFlagToSet -> Inter_Trial_State : after(2, e_clk)
  Main_Trial -> WaitForFlagToSet : e_ExitTrialNow/
      | instruct_tgt_state = 0;
      | hand_tgt_state = 0;
      | logging_enable = 0;
      | tickCount = 10;
  (junction 111) -> Inter_Trial_State : after(ITI, e_clk)
  data: forcehist function_input double size=[200,1]; itrial function_input double; meanmvc function_output double; itrial1 function_output double; force function_input double; forcehist1 function_output double size=[200,1]; currMVC function_input double; currForce function_input double; newMVC function_output double; newcount function_output double; currcount function_input double; imvc function_input double; imvc1 function_output double; max_mvc function_input double; newmax_mvc function_output double; minforce function_input double; logging_enable output boolean; event_code output double; avg_mvc_joint output double; mvc_joint local double; duration output double; hand_tgt_row output [1..32]; hand_tgt_state output double; currforce output double; tickCount local double; Trial_Protocol input double; taskbtn input double; max_move_time local double size=1; joint_force input double; target_bar_state output double; goal_force_pct output double; TrialType output double; hand_pos input double size=2; TaskWideParams input double size=50; instruct_tgt_row output double; instruct_tgt_state output double; n_mvc local double; tmp_forcehist local double size=[200,1]; tmp_counter local double; iforce local double; hold_time local double; goal_force local double; maxforce local double; min_force local double; tick local double; tmpcounter local double; tmpforce local double; ITI local double; HandInTarget input double; force_thresh local double; RepeatTrial output double; tone output double
  data hand_tgt_row settings: description=index of the row currently being used in the TargetTable
  events: e_btn input EITHER_EDGE_EVENT; e_start output EITHER_EDGE_EVENT; e_clk input RISING_EDGE_EVENT; e_ExitTrialNow input EITHER_EDGE_EVENT; e_Trial_End output EITHER_EDGE_EVENT
  function [meanmvc,itrial1,forcehist1] = calcmvc(forcehist,itrial,force):
    | function [meanmvc,itrial1,forcehist1] = calcmvc(forcehist,itrial,force)
    |  
    |  
    | itrial1 = itrial+1;
    | if itrial1 > length(forcehist)
    |     itrial1 = 1;
    | end
    | 
    | forcehist(itrial1) = force;
    | 
    | meanmvc = sum(forcehist)/sum(forcehist>0);
    | 
    | %meanmvc = mean(nonzeros(forcehist));
    | 
    | forcehist1 = forcehist;
  function [newMVC,newcount, imvc1, newmax_mvc] = update_mvc(currMVC,currForce, currcount, imvc, max_mvc, minforce):
    | function [newMVC,newcount, imvc1, newmax_mvc] = update_mvc(currMVC,currForce, currcount, imvc, max_mvc, minforce)
    | 
    | meanmvc = mean(currMVC);
    | newMVC = currMVC;
    | 
    | forcethresh = minforce;
    | 
    | %keep a running history of applied forces
    | imvc1 = imvc+1;
    | if imvc1 > length(newMVC)
    |     imvc1 = 1;
    | end
    | 
    | newMVC(imvc1) = currForce;
    | 
    | if (currForce-meanmvc) > forcethresh  %current force is greater than the current average recorded force
    |     newcount = 0;
    |     newmax_mvc = meanmvc;
    | elseif abs(currForce-meanmvc) < forcethresh %current force is within range of current average recorded force
    |     newcount = currcount+1;
    |     newmax_mvc = meanmvc;
    | else %current force is less than range of current average recorded force
    |     newcount = 0;
    |     newmax_mvc = max_mvc;
    | end

== matlab function CML_Iso_Force_Production/Trajectory subsystem/calculate robot scaling/MATLAB Function ==
  data: robot_type input; scaling output; exo_scaling input
function scaling = fcn(robot_type, exo_scaling)
%#codegen

scaling = [0, 0];

%0 = EXO, 1 = EP, 2 = NHP
for n=1:2
    if robot_type(n) == 1
        scaling(n) = 0;
    else
        scaling(n) = exo_scaling(n);
    end
end

== matlab function CML_Iso_Force_Production/Trajectory subsystem/Create_Trajectory/Virtual_Trajectory/Extract_Position ==
  settings: fimath=|
      | fimath(...
      | 'RoundMode', 'floor',...
      | 'OverflowMode', 'wrap',...
      | 'ProductMode', 'KeepLSB', 'ProductWordLength', 32,...
      | 'SumMode', 'KeepLSB', 'SumWordLength', 32,...
      | 'CastBeforeSum', false)
  data: u input; position output
function position = fcn(u)

position=[0,0];	%initialization
if length(u)==2	%input is assumed to be (x,y) position, global coordinates, (m)		
	position=u;
else			%input is assumed to be a VCODE
	position(1)=u(3);
	position(2)=u(4);
end

== matlab function CML_Iso_Force_Production/Trajectory subsystem/Create_Trajectory/Virtual_Trajectory/Extract_Position1 ==
  settings: fimath=|
      | fimath(...
      | 'RoundMode', 'floor',...
      | 'OverflowMode', 'wrap',...
      | 'ProductMode', 'KeepLSB', 'ProductWordLength', 32,...
      | 'SumMode', 'KeepLSB', 'SumWordLength', 32,...
      | 'CastBeforeSum', false)
  data: u input; position output
function position = fcn(u)

position=[0,0];	%initialization
if length(u)==2	%input is assumed to be (x,y) position, global coordinates, (m)		
	position=u;
else			%input is assumed to be a VCODE
	position(1)=u(3);
	position(2)=u(4);
end

== matlab function CML_Iso_Force_Production/Force_Fdbk_Bar/MakeBar ==
  data: currforce input; VCODES output; mvc input; goalforce input; VCODE input; heightratio output
function [VCODES,heightratio] = fcn(currforce,mvc,goalforce,VCODE)
%#codegen

%calculate the height ratio to scale the inner bar by
heightratio = currforce/mvc;

%duplicate the rectangle shape; VCODE(2,:) will be the inner fill bar,
% VCODE(1,:) will be the outer border, and VCODE(3,:) will be the goal line
VCODES = [VCODE; VCODE; VCODE];



%VCODE(1,:) specifies a fill color and no stroke color; we want to make the
%outline have no fill and a white border
VCODES(2,7) = 0; %remove the stroke width on the inner bar
VCODES(2,10) = VCODES(2,10)*.9; %shrink the width of the inner bar to fill the frame
VCODES(1,5) = createcolor(0,0,0); %set the outer frame fill to black
VCODES(1,6) = createcolor(100,100,100); %set the outer frame stroke to white

%the rectangle has dims (10,11,12) = width (x dir), height (y dir), rot
%we want to scale the inner rect height by the heightratio
VCODES(2,11) = VCODES(2,11)*heightratio;
%we need to edit the y position of the inner bar to keep the base fixed at
%the bottom of the outer frame, by subtracting half the height difference
%between the two bars
VCODES(2,4) = VCODES(2,4) - ( VCODES(1,11) - VCODES(2,11) )/2;  



%we need to add in a line representing the target height.
VCODES(3,1) = 4; %set this to be a line segment

framewidth = VCODES(1,10);
framecenterx = VCODES(1,3);
framesidex = framecenterx - framewidth/2;

frameheight = VCODES(1,11);
framebottom_pos = VCODES(1,4)-(frameheight/2);
goaloffset = frameheight*(goalforce/100);

VCODES(3,3) = framesidex;
VCODES(3,4) = framebottom_pos+goaloffset;
VCODES(3,10) = framewidth;
VCODES(3,11) = 0;
VCODES(3,6) = createcolor(100,0,0);  %set the goal color to be red

end


function color_value = createcolor(red, green, blue)
% CREATE_COLOR Given percentages of red, green and blue creates an RGB color.
% c = CREATE_COLOR(0, 100, 0) creates a pure green
% c = CREATE_COLOR(20, 0, 20) creates a dark magenta.

    red = bound(red);
    green = bound(green);
    blue = bound(blue);
    
    %convert to RGB bytes
    r = uint32(255 * (red / 100));
    g = uint32(255 * (green / 100));
    b = uint32(255 * (blue / 100));
    
    color_value = bitshift(r, 16) + bitshift(g, 8) + b;
    
end


function color = bound(c)
color = c;
if color < 0 || color > 100
    warning 'Valid values are 0-100'
    if color < 0
        color = 0;
    else
        color = 100;
    end
end
end

== matlab function CML_Iso_Force_Production/Force_Fdbk_Bar/ForceFdbk ==
  data: MVC input; CurrForce input; VCODE_mod output; VCODE input; TrialType input
function VCODE_mod  = fcn(MVC, CurrForce, VCODE, TrialType)
%#codegen

%VCODE_mod = VCODE;


%translate the current (avg) MVC to text
force_whole = int32(floor(double(MVC)));
if (force_whole >= 10) %double digit dollar value
    n1d = int32(floor(double(force_whole)/10));
    n2d = force_whole - n1d*10;
    textwhole = [int2char(int32(n1d)) int2char(int32(n2d))];
else %single digit
    textwhole = int2char(int32(force_whole));
end

force_frac = (MVC-double(force_whole))*100;
if (force_frac < 10)
    textfrac = ['0' int2char(int32(force_frac))];
else
    n1 = int32(floor(double(force_frac)/10));
    n2 = round(force_frac - n1*10);
    textfrac = [int2char(int32(n1)) int2char(int32(n2))];
end

%need to translate text into ascii:
textmvc = [double(textwhole) 46 double(textfrac)];



%translate the current force to text
force_whole = int32(floor(double(CurrForce)));
if (force_whole >= 10) %double digit dollar value
    n1d = int32(floor(double(force_whole)/10));
    n2d = force_whole - n1d*10;
    textwhole = [int2char(int32(n1d)) int2char(int32(n2d))];
else %single digit
    textwhole = int2char(int32(force_whole));
end

force_frac = (CurrForce-double(force_whole))*100;
if (force_frac < 10)
    textfrac = ['0' int2char(int32(force_frac))];
else
    n1 = int32(floor(double(force_frac)/10));
    n2 = round(force_frac - n1*10);
    textfrac = [int2char(int32(n1)) int2char(int32(n2))];
end

%need to translate text into ascii:
textcforce = [double(textwhole) 46 double(textfrac)];


textslash = ' / ';
textslash = double(char(textslash));


%set where to display the text (both screens for MVC trial, operator
%  screen only for test trial)
if TrialType == 1  %MVC trial, display the current force to the subject and both current force and average mvc to the operator
    VCODE(1,2) = 2;     %display on both screens
    
    textout = [textcforce 0];
    
    VCODE(1,15:min([15+length(textout)-1,64])) = textout(1:min([length(textout),50])); %write out as many the characters as possible into the VCODE
    VCODE(1,min([15+length(textout)+1,64])) = 0;  %terminate the string!

    VCODE_mod = [VCODE; VCODE];
    
    VCODE_mod(2,2) = 3;
    
    textout = [textcforce textslash textmvc 0];
    
    VCODE_mod(2,15:min([15+length(textout)-1,64])) = textout(1:min([length(textout),50])); %write out as many the characters as possible into the VCODE
    VCODE_mod(2,min([15+length(textout)+1,64])) = 0;  %terminate the string!


elseif TrialType == 2  %production trial; display current and MVC to the operator
    
    VCODE(1,2) = 3;   %display curent and mvc forces only to the operator
    
    textout = [textcforce textslash textmvc 0];
    
    VCODE(1,15:min([15+length(textout)-1,64])) = textout(1:min([length(textout),50])); %write out as many the characters as possible into the VCODE
    VCODE(1,min([15+length(textout)+1,64])) = 0;  %terminate the string!
    
    VCODE_mod = [VCODE; zeros(size(VCODE))];
   
else
    
    VCODE_mod = [VCODE; zeros(size(VCODE))];
    
end









function s = int2char(n)

n = mod(n,10); %make sure we only have 1 digit or we will get a weird character!

s = char(n+int32('0')); %// add the character

== stateflow chart CML_Iso_Force_Production/Trajectory subsystem/Create_Trajectory/Virtual_Trajectory/VirtualTrajectory ==
  state Initialization/
    virt_pos = reset_pos;
    // this initialization ensures that the virtual position
    // starts off as something reasonable
    traj_status = 0;   // initialize trajectory status
  state main/
    state wait_for_trigger/
      reset_controller = 0;
    state wait_1_ms_b/
      // wait for controller
      // to be reset
    state on_ramp/
      entry: tick = 0;    // initialize the tick counter
      reset_controller = 0;
      final_pos = target_pos;   // set the final position of the trajectory
      start_pos = virt_pos;   // set the start position of the trajectory
      duration = input_duration;   // store the duration of the trajectory
      traj_status = 1;   // indicate an ongoing trajectory
      during:
      on e_clk: tick++;
      // the trajectory velocity will have a bell shaped profile
      trajectory_shape = tick/duration-sin(2*pi*tick/duration)/(2*pi);
      virt_pos[1] = start_pos[1] + (final_pos[1] - start_pos[1]) * trajectory_shape;
      virt_pos[2] = start_pos[2] + (final_pos[2] - start_pos[2]) * trajectory_shape;
    main -> wait_1_ms_b [order 1] : [(robot_enabled == 1) && (traj_status == -1)]/
        | traj_status = 1;
        | virt_pos = reset_pos;
        | reset_controller = 1;
        | // trajectory was halted and
        | //is now being re-started
    wait_for_trigger -> (junction 20) : e_start
    (junction 20) -> wait_for_trigger [order 2]
    wait_1_ms_b -> (junction 20) : after(1, e_clk)
    (junction 20) -> on_ramp [order 1] : [input_duration>0]
    on_ramp -> wait_for_trigger [order 2] : [robot_enabled == 0]/
        | traj_status = -1;
        | // robot disabled
    on_ramp -> wait_for_trigger [order 1] : after(duration, e_clk)/
        | traj_status = 0
        | // trajectory completed
  state wait_1_ms/
    // wait for controller
    // to be reset
  state task_not_running/
    // wait for task_status to change
    // keep updating virt_pos so that the feedback
    // controller output, which is filtered, does not become
    // huge, resulting in a 'bump' if we don't do this.
    traj_status = 0;
    reset_controller = 0;
    during:
    virt_pos = reset_pos;
  (default) -> Initialization
  Initialization -> wait_for_trigger
  wait_1_ms -> wait_for_trigger : after(1, e_clk)
  task_not_running -> wait_1_ms : [task_status > 0]/
      | reset_controller = 1;
      | // task is running again,
      | // so reset position controller
  main -> task_not_running [order 1] : [task_status == 0]/
      | // means that run_status == 0
      | // AND that torque scaling at
      | // end of task is finished
  data: input_duration input double; target_pos input double size=[1 2]; tick local double; duration local double; reset_pos input double size=[1 2]; task_status input double; pi constant double =3.14159265358979; trajectory_shape local double; virt_pos output double size=[1 2]; traj_status output double; robot_enabled input double; start_pos local double size=[1 2]; final_pos local double size=[1 2]; reset_controller output double
  events: e_clk input RISING_EDGE_EVENT; e_start input RISING_EDGE_EVENT

== matlab function CML_Iso_Force_Production/Trajectory subsystem/Create_Trajectory/get_arm_info ==
  settings: fimath=|
      | fimath(...
      | 'RoundMode', 'floor',...
      | 'OverflowMode', 'wrap',...
      | 'ProductMode', 'KeepLSB', 'ProductWordLength', 32,...
      | 'SumMode', 'KeepLSB', 'SumWordLength', 32,...
      | 'CastBeforeSum', false)
  data: position output; task_status output; use_dom_hand input; kinarm_data input; run_status input; scaling input; robot_enabled output
function [position, task_status, robot_enabled]  = fcn(use_dom_hand, kinarm_data, run_status, scaling)
%
% get current hand position and robot enabled status
%
% May 2009
%

hpx_index = 23;
hpy_index = 24;
robot_disabled_index = 37;

%determine which arm to apply the load to
dominant_hand=kinarm_data(3,1);						%kinarm_data(3,1) tells which arm is the dominant arm
if use_dom_hand == 1
	feedback_arm = dominant_hand;
else
	feedback_arm = 3 - dominant_hand;
end

hpx = kinarm_data( feedback_arm, hpx_index );
hpy = kinarm_data( feedback_arm, hpy_index );
position = [hpx hpy];

if kinarm_data( feedback_arm, robot_disabled_index ) == 0;
    robot_enabled = 1;
else
    robot_enabled = 0;
end

% if the task has stopped/paused (i.e. run_status == 0) AND the torques outputs
% have scaled down to 0, then set the task_status = 0.
if run_status == 0 && scaling(feedback_arm) == 0
    task_status = 0;
else
    task_status = 1;
end

== matlab function CML_Iso_Force_Production/Force_Fdbk_Bar/InstructText ==
  data: MVCtrial input; goal_force input; dofdbk input; VCODE input; VCODE_mod output; instr_state input
function VCODE_mod  = fcn(MVCtrial, goal_force, dofdbk, VCODE, instr_state)
%#codegen

VCODE_mod = VCODE;

if MVCtrial == 0 && instr_state == 1 %if test trial and intsructing flex, modify instructions

    textout = [];
    
    if dofdbk == 1
        
        instruct1 = 'Flex your triceps to ';
        instruct2 = '% (reach the line).';
    else %if dofdbk == 0
        
        instruct1 = 'Flex your triceps to ';
        instruct2 = '%.';
    end
    
    %translate the goal force to text
    force_whole = int32(floor(double(goal_force)));
    if (force_whole >= 10) %double digit dollar value
        n1d = int32(floor(double(force_whole)/10));
        n2d = force_whole - n1d*10;
        textwhole = [int2char(int32(n1d)) int2char(int32(n2d))];
    else %single digit
        textwhole = int2char(int32(force_whole));
    end
    
    force_frac = (goal_force-double(force_whole))*100;
    if (force_frac < 10)
        textfrac = ['0' int2char(int32(force_frac))];
    else
        n1 = int32(floor(double(force_frac)/10));
        n2 = round(force_frac - n1*10);
        textfrac = [int2char(int32(n1)) int2char(int32(n2))];
    end
    
    %need to translate text into ascii:
    if force_frac < 1 %no fractional percentage
        textforce = [double(textwhole)];
    else %some fractional percentage
        textforce = [double(textwhole) 46 double(textfrac)];
    end
    
    textout = [double(instruct1) textforce double(instruct2) 0];
    


    VCODE_mod(1,15:min([15+length(textout)-1,64])) = textout(1:min([length(textout),50])); %write out as many the characters as possible into the VCODE
    VCODE_mod(1,min([15+length(textout)+1,64])) = 0;  %terminate the string!

end






function s = int2char(n)

n = mod(n,10); %make sure we only have 1 digit or we will get a weird character!

s = char(n+int32('0')); %// add the character

== matlab function CML_Iso_Force_Production/Play Sound/Play sound over and over ==
  data: tone input; output output; beep input; errorbeep input; coin input
function output = fcn(tone,beep,errorbeep,coin)
%#codegen

persistent t last_tone_state
if isempty(t), t = 0; end
if isempty(last_tone_state), last_tone_state = 0; end

trigger = last_tone_state ~= tone;
if trigger > 0
    last_tone_state = tone;
end

output = 0;		% default
if t == 0 && trigger > 0
	% start the playing of the sound.
	t = t + 1;
end

if tone == 1
    data = beep;
elseif tone == 2
    data = coin;
elseif tone == 3
    data = errorbeep;
else 
    t = 0;
    data = 0;
end

if t > 0
	output = data(t);
	if t == length(data)
		t = 0;
	else
		t = t + 1;
	end
end
